simulink model "Model_3"  (R2020b)
settings: Solver=ode45  StartTime=0.0  StopTime=120  RelTol=1e-3
values from neighbouring files (symbols this model uses):
  b = 50    [Variables.m]
  M = 1000    [Variables.m]
settings Model: Creator=samar  LastModifiedBy=samar

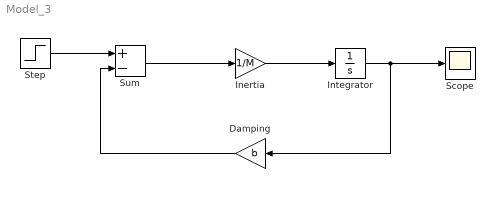
== system Model_3 ==
  Damping : Gain  Gain=b
  Inertia : Gain  Gain=1/M
  Integrator : Integrator
  Scope : Scope
  Step : Step  After=u  SampleTime=0
  Sum : Sum  Inputs=+-
  wires:
  Step/1 -> Sum/1
  Sum/1 -> Inertia/1
  Inertia/1 -> Integrator/1
  Integrator/1 -> Damping/1, Scope/1
  Damping/1 -> Sum/2
